simulink model "segway_control"  (R2022a)
settings: Solver=ode45  StartTime=0.0  StopTime=30  FixedStep=1e-3  RelTol=1e-3
PreLoadFcn:
  | preload
InitFcn:
  | init
  | preload
values from neighbouring files (symbols this model uses):
  A1 = [0 0   1 0 ... (first row only)    [plant.m]
  A2 = [0   1 ... (first row only)    [plant.m]
  B1 = [0 0 ... (first row only)    [plant.m]
  B2 = [0    0 ... (first row only)    [plant.m]
  C1 = [1 0 0 0 ... (first row only)    [plant.m]
  C2 = [1 0 ... (first row only)    [plant.m]
  D = 0.01    [params.m]
  D1 = zeros(4, 2)    [plant.m]
  D2 = zeros(2)    [plant.m]
  h = 0.21    [params.m]
  Jw = m * R^2 / 2    (= 0.0001458)    [params.m]
  Jwx = m * (3*R^2 + hw^2) / 12    (= 8.62333333333e-05)    [params.m]
  K = lqrd(s4.A, s4.B, QQ, RR, Ts)    [control.m]    (also in plant.m = W / (2 * R) * alpha)
  K_PWM = 8.087    [params.m]
  Kb = 0.468    [params.m]
  Kt = 0.317    [params.m]
  Lm = 0.0029    [params.m]
  m = 0.4    [params.m]
  M = 1.8    [params.m]
  R = 0.027    [params.m]
  Rm = 6.69    [params.m]
  W = 0.105    [params.m]
undefined symbols (not defined in the file or in its folder): X, Y, Z
libraries: sm_lib x17, nesl_utility x13, simulink_extras x7
settings Model: Creator=skakd  LastModifiedBy=skakd
settings SolverCC: ZeroCrossControl=EnableAll  ZeroCrossAlgorithm=Adaptive  EnableFixedStepZeroCrossing=on

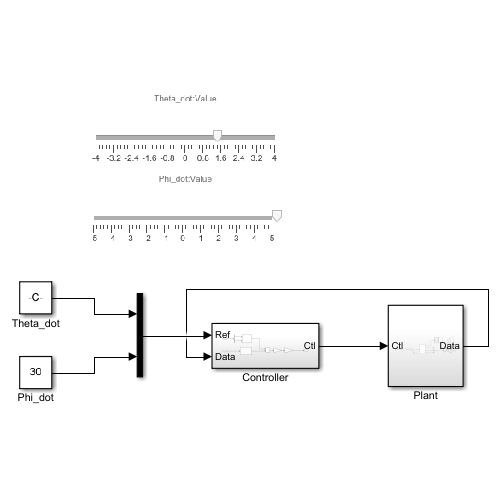
[thumbnail: Simulink's stored preview of the top-level diagram]
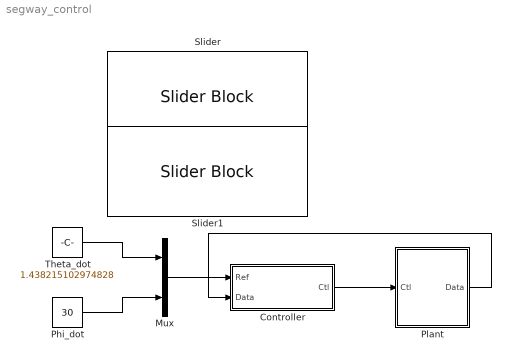
== system segway_control ==
  Controller : Subsystem
  Mux : Mux  Inputs=2
  Phi_dot : Constant  Value=30
  Plant : Subsystem
  Slider : SliderBlock  ScaleMin=-4  ScaleMax=4
  Slider1 : SliderBlock  ScaleMin=-5  ScaleMax=5
  Theta_dot : Constant  Value=1.438215102974828
  wires:
  Theta_dot/1 -> Mux/1
  Phi_dot/1 -> Mux/2
  Mux/1 -> Controller/1(Ref)
  Controller/1(Ctl) -> Plant/1(Ctl)
  Plant/1(Data) -> Controller/2(Data)

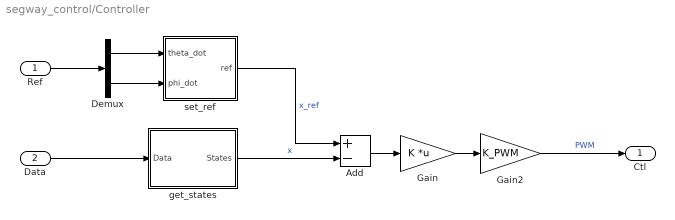
== system segway_control/Controller ==
  Ref : Inport
  Data : Inport  Port=2
  Add : Sum  Inputs=+-
  Demux : Demux  Outputs=2
  Gain : Gain  Gain=K  Multiplication=Matrix(K*u)
  Gain2 : Gain  Gain=K_PWM
  get_states : Subsystem
  set_ref : Subsystem
  Ctl : Outport  VectorParamsAs1DForOutWhenUnconnected=off
  wires:
  Gain2/1 -> Ctl/1  "PWM"
  Add/1 -> Gain/1
  set_ref/1(ref) -> Add/1  "x_ref"
  Gain/1 -> Gain2/1
  Ref/1 -> Demux/1
  Demux/1 -> set_ref/1(theta_dot)
  Demux/2 -> set_ref/2(phi_dot)
  get_states/1(States) -> Add/2  "x"
  Data/1 -> get_states/1(Data)

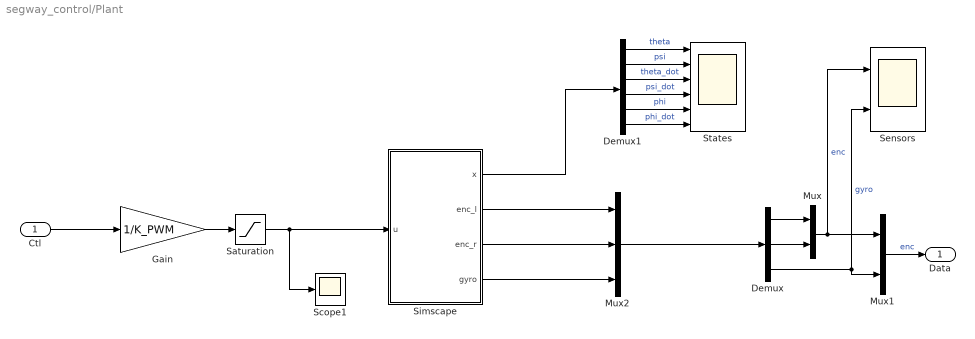
== system segway_control/Plant ==
  Ctl : Inport
  Demux : Demux  Outputs=3
  Demux1 : Demux  Outputs=6
  Gain : Gain  Gain=1/K_PWM
  Mux : Mux  Inputs=2
  Mux1 : Mux  Inputs=2
  Mux2 : Mux  Inputs=3
  Saturation : Saturate  UpperLimit=80  LowerLimit=-80
  Scope1 : Scope
  Sensors : Scope  NumInputPorts=2
  Simscape : Subsystem  Variant=on  VariantControl=Choice
  States : Scope  NumInputPorts=6
  Data : Outport
  wires:
  Mux2/1 -> Demux/1
  Demux/1 -> Mux/1
  Demux/2 -> Mux/2
  Mux/1 -> Mux1/1, Sensors/1  "enc"
  Demux/3 -> Mux1/2, Sensors/2  "gyro"
  Ctl/1 -> Gain/1
  Demux1/3 -> States/3  "theta_dot"
  Demux1/1 -> States/1  "theta"
  Demux1/4 -> States/4  "psi_dot"
  Demux1/6 -> States/6  "phi_dot"
  Demux1/2 -> States/2  "psi"
  Demux1/5 -> States/5  "phi"
  Gain/1 -> Saturation/1
  Saturation/1 -> Scope1/1, Simscape/1(u)
  Simscape/1(x) -> Demux1/1
  Simscape/2(enc_l) -> Mux2/1
  Simscape/3(enc_r) -> Mux2/2
  Simscape/4(gyro) -> Mux2/3
  Mux1/1 -> Data/1  "enc"

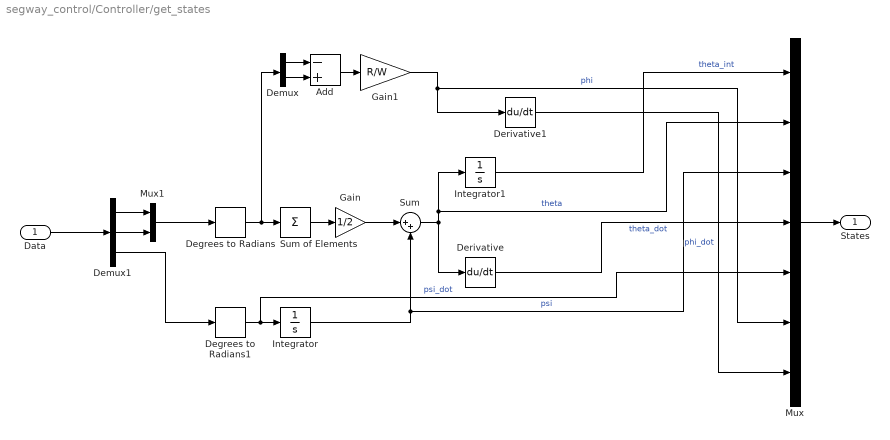
== system segway_control/Controller/get_states ==
  Data : Inport
  Add : Sum  Inputs=-+
  Degrees to Radians : simulink_extras/Transformations/Degrees to Radians
  Degrees to Radians1 : simulink_extras/Transformations/Degrees to Radians
  Demux : Demux  Outputs=2
  Demux1 : Demux  Outputs=3
  Derivative : Derivative
  Derivative1 : Derivative
  Gain : Gain  Gain=1/2
  Gain1 : Gain  Gain=R/W
  Integrator : Integrator
  Integrator1 : Integrator
  Mux : Mux  Inputs=7
  Mux1 : Mux  Inputs=2
  Sum : Sum  Inputs=|++
  Sum of Elements : Sum  Inputs=+
  States : Outport  VectorParamsAs1DForOutWhenUnconnected=off
  wires:
  Gain/1 -> Sum/1
  Degrees to Radians/1 -> Demux/1, Sum of Elements/1
  Integrator/1 -> Mux/3, Sum/2  "psi"
  Data/1 -> Demux1/1
  Mux1/1 -> Degrees to Radians/1
  Sum/1 -> Mux/2, Integrator1/1, Derivative/1  "theta"
  Derivative/1 -> Mux/4  "theta_dot"
  Sum of Elements/1 -> Gain/1
  Degrees to Radians1/1 -> Mux/5, Integrator/1  "psi_dot"
  Integrator1/1 -> Mux/1  "theta_int"
  Demux/1 -> Add/1
  Demux/2 -> Add/2
  Add/1 -> Gain1/1
  Gain1/1 -> Mux/6, Derivative1/1  "phi"
  Derivative1/1 -> Mux/7  "phi_dot"
  Mux/1 -> States/1
  Demux1/1 -> Mux1/1
  Demux1/2 -> Mux1/2
  Demux1/3 -> Degrees to Radians1/1

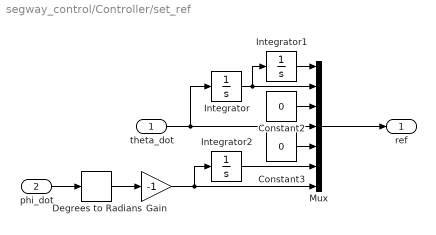
== system segway_control/Controller/set_ref ==
  theta_dot : Inport
  phi_dot : Inport  Port=2
  Constant2 : Constant  Value=0
  Constant3 : Constant  Value=0
  Degrees to Radians : simulink_extras/Transformations/Degrees to Radians
  Gain : Gain  Gain=-1
  Integrator : Integrator
  Integrator1 : Integrator
  Integrator2 : Integrator
  Mux : Mux  Inputs=7
  ref : Outport  VectorParamsAs1DForOutWhenUnconnected=off
  wires:
  Constant2/1 -> Mux/3
  Constant3/1 -> Mux/5
  Mux/1 -> ref/1
  Integrator/1 -> Integrator1/1, Mux/2
  phi_dot/1 -> Degrees to Radians/1
  Integrator2/1 -> Mux/6
  Integrator1/1 -> Mux/1
  theta_dot/1 -> Integrator/1, Mux/4
  Degrees to Radians/1 -> Gain/1
  Gain/1 -> Integrator2/1, Mux/7

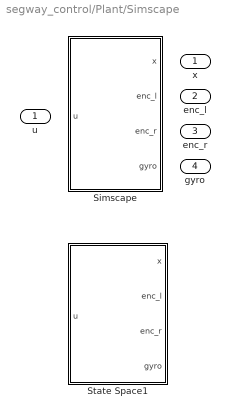
== system segway_control/Plant/Simscape ==
  u : Inport
  Simscape : Subsystem  VariantControl=(default)
  State Space1 : Subsystem  VariantControl=is_simscape == 0
  x : Outport
  enc_l : Outport  Port=2
  enc_r : Outport  Port=3
  gyro : Outport  Port=4

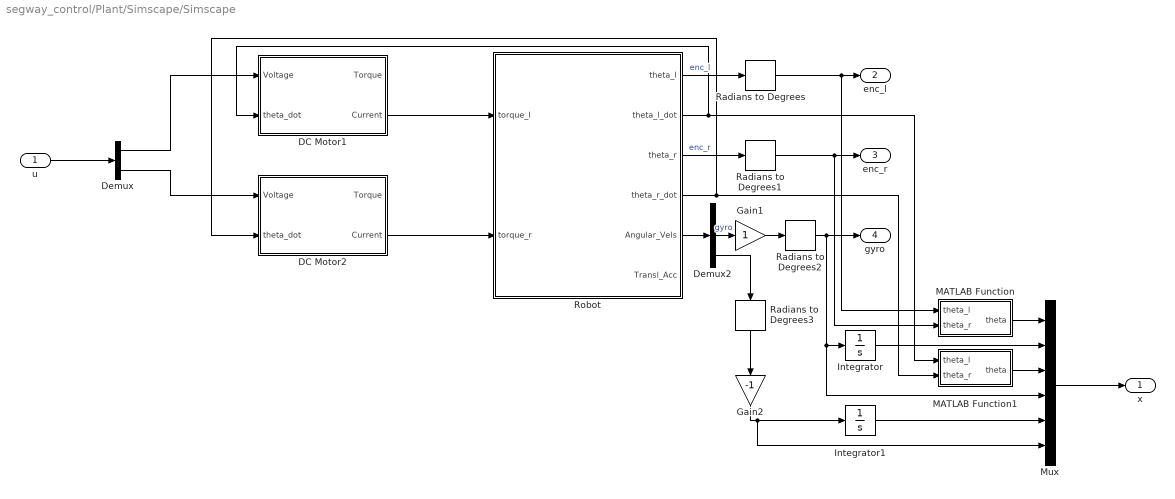
== system segway_control/Plant/Simscape/Simscape ==
  u : Inport
  DC Motor1 : Subsystem
  DC Motor2 : Subsystem
  Demux : Demux  Outputs=2
  Demux2 : Demux  Outputs=3
  Gain1 : Gain
  Gain2 : Gain  Gain=-1
  Integrator : Integrator
  Integrator1 : Integrator
  MATLAB Function : MATLAB Function  TreatAsAtomicUnit=on
  MATLAB Function1 : MATLAB Function  TreatAsAtomicUnit=on
  Mux : Mux  Inputs=6
  Radians to Degrees{,1..3} (4 alike) : simulink_extras/Transformations/Radians to Degrees
  Robot : Subsystem
  x : Outport
  enc_l : Outport  Port=2
  enc_r : Outport  Port=3
  gyro : Outport  Port=4
  wires:
  Robot/5(Angular_Vels) -> Demux2/1
  Demux2/2 -> Gain1/1  "gyro"
  Radians to Degrees1/1 -> MATLAB Function/2(theta_r), enc_r/1
  Robot/3(theta_r) -> Radians to Degrees1/1  "enc_r"
  Radians to Degrees/1 -> MATLAB Function/1(theta_l), enc_l/1
  Robot/1(theta_l) -> Radians to Degrees/1  "enc_l"
  Radians to Degrees2/1 -> gyro/1, Mux/4, Integrator/1
  u/1 -> Demux/1
  Mux/1 -> x/1
  Integrator/1 -> Mux/2
  Demux2/3 -> Radians to Degrees3/1
  Integrator1/1 -> Mux/5
  MATLAB Function/1(theta) -> Mux/1
  MATLAB Function1/1(theta) -> Mux/3
  Robot/2(theta_l_dot) -> DC Motor1/2(theta_dot), MATLAB Function1/1(theta_l)
  Robot/4(theta_r_dot) -> DC Motor2/2(theta_dot), MATLAB Function1/2(theta_r)
  Gain1/1 -> Radians to Degrees2/1
  Demux/1 -> DC Motor1/1(Voltage)
  Demux/2 -> DC Motor2/1(Voltage)
  Gain2/1 -> Integrator1/1, Mux/6
  DC Motor1/2(Current) -> Robot/1(torque_l)
  DC Motor2/2(Current) -> Robot/2(torque_r)
  Radians to Degrees3/1 -> Gain2/1

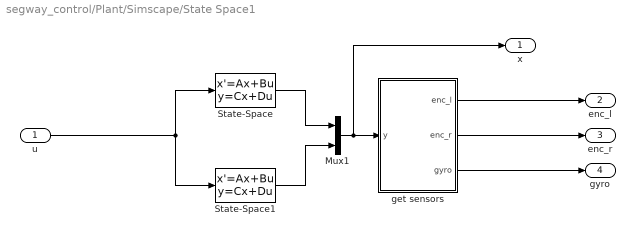
== system segway_control/Plant/Simscape/State Space1 ==
  u : Inport
  Mux1 : Mux  Inputs=2
  State-Space : StateSpace  A=A1  B=B1  C=C1  D=D1  InitialCondition=0
  State-Space1 : StateSpace  A=A2  B=B2  C=C2  D=D2  InitialCondition=0
  get sensors : MATLAB Function  TreatAsAtomicUnit=on
  x : Outport
  enc_l : Outport  Port=2
  enc_r : Outport  Port=3
  gyro : Outport  Port=4
  wires:
  get sensors/3(gyro) -> gyro/1
  get sensors/2(enc_r) -> enc_r/1
  State-Space1/1 -> Mux1/2
  u/1 -> State-Space1/1, State-Space/1
  Mux1/1 -> get sensors/1(y), x/1
  State-Space/1 -> Mux1/1
  get sensors/1(enc_l) -> enc_l/1

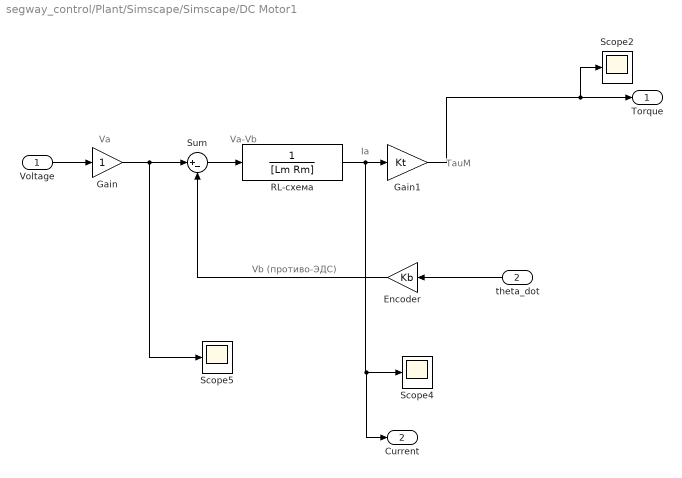
== system segway_control/Plant/Simscape/Simscape/DC Motor1 ==
  note: Va
  note: Va-Vb
  note: Vb (противо-ЭДС)
  note: Ia
  note: TauM
  Voltage : Inport
  theta_dot : Inport  Port=2
  Encoder : Gain  Gain=Kb
  Gain : Gain
  Gain1 : Gain  Gain=Kt
  RL-схема : TransferFcn  Denominator=[Lm Rm]
  Scope2 : Scope
  Scope4 : Scope
  Scope5 : Scope
  Sum : Sum  Inputs=|+-
  Torque : Outport
  Current : Outport  Port=2
  wires:
  Voltage/1 -> Gain/1
  Encoder/1 -> Sum/2
  Sum/1 -> RL-схема/1
  RL-схема/1 -> Gain1/1, Scope4/1, Current/1
  Gain/1 -> Sum/1, Scope5/1
  Gain1/1 -> Scope2/1, Torque/1
  theta_dot/1 -> Encoder/1

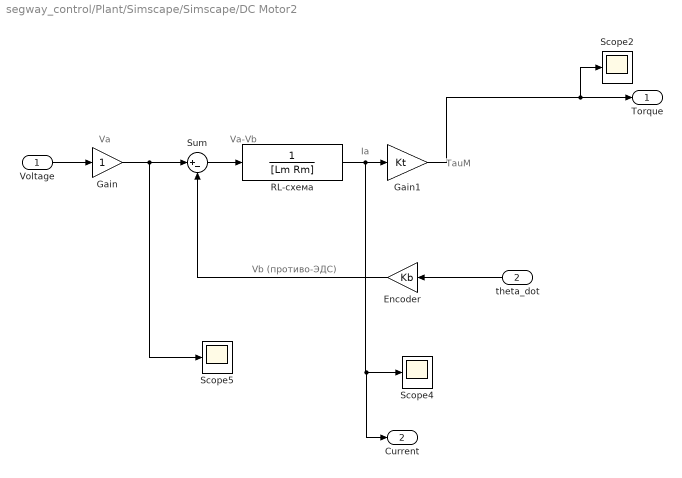
== system segway_control/Plant/Simscape/Simscape/DC Motor2 ==
  note: TauM
  note: Ia
  note: Vb (противо-ЭДС)
  note: Va-Vb
  note: Va
  Voltage : Inport
  theta_dot : Inport  Port=2
  Encoder : Gain  Gain=Kb
  Gain : Gain
  Gain1 : Gain  Gain=Kt
  RL-схема : TransferFcn  Denominator=[Lm Rm]
  Scope2 : Scope
  Scope4 : Scope
  Scope5 : Scope
  Sum : Sum  Inputs=|+-
  Torque : Outport
  Current : Outport  Port=2
  wires:
  theta_dot/1 -> Encoder/1
  Gain1/1 -> Torque/1, Scope2/1
  Gain/1 -> Scope5/1, Sum/1
  RL-схема/1 -> Current/1, Scope4/1, Gain1/1
  Sum/1 -> RL-схема/1
  Encoder/1 -> Sum/2
  Voltage/1 -> Gain/1

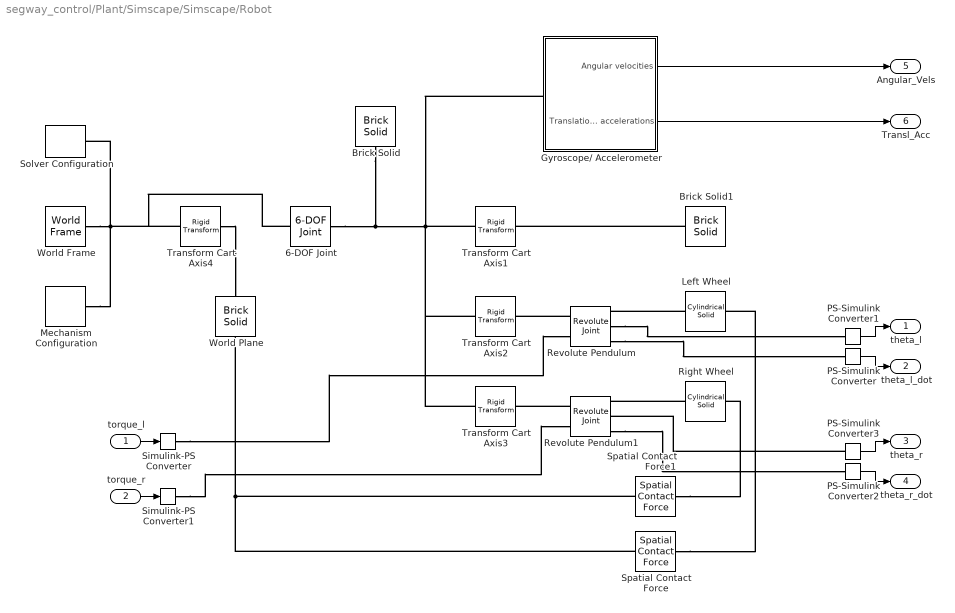
== system segway_control/Plant/Simscape/Simscape/Robot ==
  torque_l : Inport
  torque_r : Inport  Port=2
  6-DOF Joint : sm_lib/Joints/6-DOF Joint  JointMode=Normal  SenseConstraintForce=off  SenseConstraintForceX=off  SenseConstraintForceY=off  SenseConstraintForceZ=off  SenseConstraintTorque=off  SenseConstraintTorqueX=off  SenseConstraintTorqueY=off  SenseConstraintTorqueZ=off  SenseTotalForce=off  SenseTotalForceX=off  SenseTotalForceY=off  SenseTotalForceZ=off  SenseTotalTorque=off  SenseTotalTorqueX=off  SenseTotalTorqueY=off  SenseTotalTorqueZ=off  CompositeWrenchDir=FollowerOnBase  CompositeWrenchFrame=BaseFrame  PxEquilibriumPosition=0  PxEquilibriumPositionUnits=m  PxSpringStiffness=0  PxSpringStiffnessUnits=N/m  PxDampingCoefficient=0  PxDampingCoefficientUnits=N/(m/s)  PxTorqueActuationMode=NoTorque  PxMotionActuationMode=ComputedMotion  PxSensePosition=off  PxSenseVelocity=off  PxSenseAcceleration=off  PxSenseTorqueForce=off  PxSenseLowerLimitTorqueForce=off  PxSenseUpperLimitTorqueForce=off  PxLowerLimitSpecify=off  PxLowerLimitBound=-1  PxLowerLimitBoundUnits=m  PxLowerLimitStiffness=1e6  PxLowerLimitStiffnessUnits=N/m  PxLowerLimitDamping=1e3  PxLowerLimitDampingUnits=N/(m/s)  PxLowerLimitTransitionRegionWidth=1e-4  PxLowerLimitTransitionRegionWidthUnits=m  PxUpperLimitSpecify=off  PxUpperLimitBound=1  PxUpperLimitBoundUnits=m  PxUpperLimitStiffness=1e6  PxUpperLimitStiffnessUnits=N/m  PxUpperLimitDamping=1e3  PxUpperLimitDampingUnits=N/(m/s)  PxUpperLimitTransitionRegionWidth=1e-4  PxUpperLimitTransitionRegionWidthUnits=m  PxPositionTargetSpecify=off  PxPositionTargetPriority=High  PxPositionTargetValue=0  PxPositionTargetValueUnits=m  PxVelocityTargetSpecify=off  PxVelocityTargetPriority=High  PxVelocityTargetValue=0  PxVelocityTargetValueUnits=m/s  PyEquilibriumPosition=0  PyEquilibriumPositionUnits=m  PySpringStiffness=0  PySpringStiffnessUnits=N/m  PyDampingCoefficient=0  PyDampingCoefficientUnits=N/(m/s)  PyTorqueActuationMode=NoTorque  PyMotionActuationMode=ComputedMotion  PySensePosition=off  PySenseVelocity=off  PySenseAcceleration=off  PySenseTorqueForce=off  PySenseLowerLimitTorqueForce=off  PySenseUpperLimitTorqueForce=off  PyLowerLimitSpecify=off  PyLowerLimitBound=-1  PyLowerLimitBoundUnits=m  PyLowerLimitStiffness=1e6  PyLowerLimitStiffnessUnits=N/m  PyLowerLimitDamping=1e3  PyLowerLimitDampingUnits=N/(m/s)  PyLowerLimitTransitionRegionWidth=1e-4  PyLowerLimitTransitionRegionWidthUnits=m  PyUpperLimitSpecify=off  PyUpperLimitBound=1  PyUpperLimitBoundUnits=m  PyUpperLimitStiffness=1e6  PyUpperLimitStiffnessUnits=N/m  PyUpperLimitDamping=1e3  PyUpperLimitDampingUnits=N/(m/s)  PyUpperLimitTransitionRegionWidth=1e-4  PyUpperLimitTransitionRegionWidthUnits=m  PyPositionTargetSpecify=off  PyPositionTargetPriority=High  PyPositionTargetValue=0  PyPositionTargetValueUnits=m  PyVelocityTargetSpecify=off  PyVelocityTargetPriority=High  PyVelocityTargetValue=0  PyVelocityTargetValueUnits=m/s  PzEquilibriumPosition=0  PzEquilibriumPositionUnits=m  PzSpringStiffness=0  PzSpringStiffnessUnits=N/m  PzDampingCoefficient=0  PzDampingCoefficientUnits=N/(m/s)  PzTorqueActuationMode=NoTorque  PzMotionActuationMode=ComputedMotion  PzSensePosition=off  PzSenseVelocity=off  PzSenseAcceleration=off  PzSenseTorqueForce=off  PzSenseLowerLimitTorqueForce=off  PzSenseUpperLimitTorqueForce=off  PzLowerLimitSpecify=off  PzLowerLimitBound=-1  PzLowerLimitBoundUnits=m  PzLowerLimitStiffness=1e6  PzLowerLimitStiffnessUnits=N/m  PzLowerLimitDamping=1e3  PzLowerLimitDampingUnits=N/(m/s)  PzLowerLimitTransitionRegionWidth=1e-4  PzLowerLimitTransitionRegionWidthUnits=m  PzUpperLimitSpecify=off  PzUpperLimitBound=1  PzUpperLimitBoundUnits=m  PzUpperLimitStiffness=1e6  PzUpperLimitStiffnessUnits=N/m  PzUpperLimitDamping=1e3  PzUpperLimitDampingUnits=N/(m/s)  PzUpperLimitTransitionRegionWidth=1e-4  PzUpperLimitTransitionRegionWidthUnits=m  PzPositionTargetSpecify=on  PzPositionTargetPriority=High  PzPositionTargetValue=R+0.025  PzPositionTargetValueUnits=m  PzVelocityTargetSpecify=off  PzVelocityTargetPriority=High  PzVelocityTargetValue=0  PzVelocityTargetValueUnits=m/s  SphDefPosRotationMethod=None  SphDefPosRotationAngleUnits=deg  SphDefPosRotationStandardAxis=+Z  SphDefPosRotationAngle=0.0  SphDefPosRotationArbitraryAxis=[0 0 1]  SphDefPosFollAlignAxisA=+X  SphDefPosBaseAlignAxisA=+Y  SphDefPosFollAlignAxisB=+Y  SphDefPosBaseAlignAxisB=+Z  SphDefPosRotationSequenceAxes=FollowerAxes  SphDefPosRotationSequence=XYX  SphDefPosRotationSequenceAngles=[0 0 0]  SphDefPosRotationSequenceAnglesUnits=deg  SphDefPosRotationMatrix=[1 0 0; 0 1 0; 0 0 1]  SphEqPosRotationMethod=None  SphEqPosRotationAngleUnits=deg  SphEqPosRotationStandardAxis=+Z  SphEqPosRotationAngle=0.0  SphEqPosRotationArbitraryAxis=[0 0 1]  SphEqPosFollAlignAxisA=+X  SphEqPosBaseAlignAxisA=+Y  SphEqPosFollAlignAxisB=+Y  SphEqPosBaseAlignAxisB=+Z  SphEqPosRotationSequenceAxes=FollowerAxes  SphEqPosRotationSequence=XYX  SphEqPosRotationSequenceAngles=[0 0 0]  SphEqPosRotationSequenceAnglesUnits=deg  SphEqPosRotationMatrix=[1 0 0; 0 1 0; 0 0 1]  SphSpringStiffness=0  SphSpringStiffnessUnits=N*m/deg  SphDampingCoefficient=0  SphDampingCoefficientUnits=N*m/(deg/s)  SphActuateTorqueX=off  SphActuateTorqueY=off  SphActuateTorqueZ=off  SphActuateTorque=off  SphTorqueActuationMode=NoTorque  SphMotionActuationMode=ComputedMotion  SphActuationFrame=BaseFrame  SphSensePosition=off  SphSenseVelocityX=off  SphSenseVelocityY=off  SphSenseVelocityZ=off  SphSenseVelocity=off  SphSenseAccelerationX=off  SphSenseAccelerationY=off  SphSenseAccelerationZ=off  SphSenseAcceleration=off  SphSenseTorqueX=off  SphSenseTorqueY=off  SphSenseTorqueZ=off  SphSenseTorqueForce=off  SphSenseLowerLimitTorqueMag=off  SphSenseUpperLimitTorqueMag=off  SphSensingFrame=BaseFrame  SphLowerLimitSpecify=off  SphLowerLimitBound=15  SphLowerLimitBoundUnits=deg  SphLowerLimitStiffness=1e4  SphLowerLimitStiffnessUnits=N*m/deg  SphLowerLimitDamping=10  SphLowerLimitDampingUnits=N*m/(deg/s)  SphLowerLimitTransitionRegionWidth=0.1  SphLowerLimitTransitionRegionWidthUnits=deg  SphUpperLimitSpecify=off  SphUpperLimitBound=45  SphUpperLimitBoundUnits=deg  SphUpperLimitStiffness=1e4  SphUpperLimitStiffnessUnits=N*m/deg  SphUpperLimitDamping=10  SphUpperLimitDampingUnits=N*m/(deg/s)  SphUpperLimitTransitionRegionWidth=0.1  SphUpperLimitTransitionRegionWidthUnits=deg  SphPositionTargetRotationMethod=None  SphPositionTargetRotationAngleUnits=deg  SphPositionTargetRotationStandardAxis=+Z  SphPositionTargetRotationAngle=0.0  SphPositionTargetRotationArbitraryAxis=[0 0 1]  SphPositionTargetFollAlignAxisA=+X  SphPositionTargetBaseAlignAxisA=+Y  SphPositionTargetFollAlignAxisB=+Y  SphPositionTargetBaseAlignAxisB=+Z  SphPositionTargetRotationSequenceAxes=FollowerAxes  SphPositionTargetRotationSequence=XYX  SphPositionTargetRotationSequenceAngles=[0 0 0]  SphPositionTargetRotationSequenceAnglesUnits=deg  SphPositionTargetRotationMatrix=[1 0 0; 0 1 0; 0 0 1]  SphPositionTargetSpecify=off  SphPositionTargetPriority=High  SphVelocityTargetValue=[0 0 0]  SphVelocityTargetValueUnits=deg/s  SphVelocityTargetSpecify=off  SphVelocityTargetPriority=High  SphVelocityTargetInFollowerFrame=on
  Brick Solid : sm_lib/Body Elements/Brick Solid  GraphicAmbientColor=[0.15 0.15 0.15 1.0]  BasedOnType=Density  BrickDimensions=[0.01 W 0.01]  BrickDimensionUnits=m  CenterOfMass=[0 0 0]  CenterOfMassUnits=m  GraphicDiffuseColor=[0.5 0.5 0.5]  Density=10  DensityUnits=kg/m^3  DoExposeReferenceFrame=on  GraphicEmissiveColor=[0.0 0.0 0.0 1.0]  ExportEntireGeometry=off  SerializedFrames=<Frames/>  MarkerShape=Sphere  MarkerSize=10  GraphicType=FromGeometry  InertiaType=CalculateFromGeometry  Mass=10  MassUnits=kg  MomentsOfInertia=[1 1 1]  MomentsOfInertiaUnits=kg*m^2  GraphicOpacity=1.0  ProductsOfInertia=[0 0 0]  ProductsOfInertiaUnits=kg*m^2  GraphicShininess=75  GraphicSpecularColor=[0.5 0.5 0.5 1.0]  GraphicVisPropType=SimpleVisualProperties
  Brick Solid1 : sm_lib/Body Elements/Brick Solid  GraphicAmbientColor=[0.15 0.15 0.15 1.0]  BasedOnType=Mass  BrickDimensions=[D W h]  BrickDimensionUnits=m  CenterOfMass=[0 0 0]  CenterOfMassUnits=m  GraphicDiffuseColor=[1.0 1.0 0.0]  Density=40000  DensityUnits=kg/m^3  DoExposeReferenceFrame=on  GraphicEmissiveColor=[0.0 0.0 0.0 1.0]  ExportEntireGeometry=on  SerializedFrames=<Frames/>  MarkerShape=Sphere  MarkerSize=10  GraphicType=FromGeometry  InertiaType=CalculateFromGeometry  Mass=M  MassUnits=kg  MomentsOfInertia=[1 1 1]  MomentsOfInertiaUnits=kg*m^2  GraphicOpacity=1.0  ProductsOfInertia=[0 0 0]  ProductsOfInertiaUnits=kg*m^2  GraphicShininess=75  GraphicSpecularColor=[0.5 0.5 0.5 1.0]  GraphicVisPropType=SimpleVisualProperties
  Gyroscope/ Accelerometer : Subsystem
  Left Wheel : sm_lib/Body Elements/Cylindrical Solid  GraphicAmbientColor=[0.15 0.15 0.15 1.0]  BasedOnType=Mass  CenterOfMass=[0 0 0]  CenterOfMassUnits=m  GraphicDiffuseColor=[0.2 0.2 0.2]  CylinderLength=0.02  CylinderLengthUnits=m  CylinderRadius=R  CylinderRadiusUnits=m  Density=5000  DensityUnits=kg/m^3  DoExposeReferenceFrame=on  GraphicEmissiveColor=[0.0 0.0 0.0 1.0]  ExportEntireGeometry=on  SerializedFrames=<Frames/>  MarkerShape=Sphere  MarkerSize=10  GraphicType=FromGeometry  InertiaType=CalculateFromGeometry  Mass=m  MassUnits=kg  MomentsOfInertia=[0 0 Jw]  MomentsOfInertiaUnits=kg*m^2  GraphicOpacity=1.0  ProductsOfInertia=[0 0 0]  ProductsOfInertiaUnits=kg*m^2  GraphicShininess=75  GraphicSpecularColor=[0.5 0.5 0.5 1.0]  GraphicVisPropType=SimpleVisualProperties
  Mechanism Configuration : sm_lib/Utilities/Mechanism Configuration  UniformGravity=Constant  GravityVector=[0 0 -9.80665]  GravityUnits=m/s^2  LinearizationDelta=0.001  JointModeTransitionNonlinearIterations=2
  PS-Simulink Converter{,1..3} (4 alike) : nesl_utility/PS-Simulink Converter  PhysicalDomain=network_engine_domain  SubClassName=ps_output  LeftPortType=input  RightPortType=output  PseudoPeriodic=off  Frequencies=[]  VectorFormat=inherit  Unit=inherit  AffineConversion=off
      settings: SourceProductBaseCode=SS,PW,VE
  Revolute Pendulum : sm_lib/Joints/Revolute Joint  JointMode=Normal  SenseConstraintForce=off  SenseConstraintForceX=off  SenseConstraintForceY=off  SenseConstraintForceZ=off  SenseConstraintTorque=off  SenseConstraintTorqueX=off  SenseConstraintTorqueY=off  SenseConstraintTorqueZ=off  SenseTotalForce=off  SenseTotalForceX=off  SenseTotalForceY=off  SenseTotalForceZ=off  SenseTotalTorque=off  SenseTotalTorqueX=off  SenseTotalTorqueY=off  SenseTotalTorqueZ=off  CompositeWrenchDir=FollowerOnBase  CompositeWrenchFrame=BaseFrame  EquilibriumPosition=0  EquilibriumPositionUnits=deg  SpringStiffness=0  SpringStiffnessUnits=N*m/deg  DampingCoefficient=fm  DampingCoefficientUnits=N*m/(deg/s)  TorqueActuationMode=InputTorque  MotionActuationMode=ComputedMotion  SensePosition=on  SenseVelocity=on  SenseAcceleration=off  SenseTorqueForce=off  SenseLowerLimitTorqueForce=off  SenseUpperLimitTorqueForce=off  LowerLimitSpecify=off  LowerLimitBound=-90  LowerLimitBoundUnits=deg  LowerLimitStiffness=1e4  LowerLimitStiffnessUnits=N*m/deg  LowerLimitDamping=10  LowerLimitDampingUnits=N*m/(deg/s)  LowerLimitTransitionRegionWidth=0.1  LowerLimitTransitionRegionWidthUnits=deg  UpperLimitSpecify=off  UpperLimitBound=90  UpperLimitBoundUnits=deg  UpperLimitStiffness=1e4  UpperLimitStiffnessUnits=N*m/deg  UpperLimitDamping=10  UpperLimitDampingUnits=N*m/(deg/s)  UpperLimitTransitionRegionWidth=0.1  UpperLimitTransitionRegionWidthUnits=deg  PositionTargetSpecify=off  PositionTargetPriority=High  PositionTargetValue=0  PositionTargetValueUnits=deg  VelocityTargetSpecify=off  VelocityTargetPriority=High  VelocityTargetValue=0  VelocityTargetValueUnits=deg/s
  Revolute Pendulum1 : sm_lib/Joints/Revolute Joint  JointMode=Normal  SenseConstraintForce=off  SenseConstraintForceX=off  SenseConstraintForceY=off  SenseConstraintForceZ=off  SenseConstraintTorque=off  SenseConstraintTorqueX=off  SenseConstraintTorqueY=off  SenseConstraintTorqueZ=off  SenseTotalForce=off  SenseTotalForceX=off  SenseTotalForceY=off  SenseTotalForceZ=off  SenseTotalTorque=off  SenseTotalTorqueX=off  SenseTotalTorqueY=off  SenseTotalTorqueZ=off  CompositeWrenchDir=FollowerOnBase  CompositeWrenchFrame=BaseFrame  EquilibriumPosition=0  EquilibriumPositionUnits=deg  SpringStiffness=0  SpringStiffnessUnits=N*m/deg  DampingCoefficient=fm  DampingCoefficientUnits=N*m/(deg/s)  TorqueActuationMode=InputTorque  MotionActuationMode=ComputedMotion  SensePosition=on  SenseVelocity=on  SenseAcceleration=off  SenseTorqueForce=off  SenseLowerLimitTorqueForce=off  SenseUpperLimitTorqueForce=off  LowerLimitSpecify=off  LowerLimitBound=-90  LowerLimitBoundUnits=deg  LowerLimitStiffness=1e4  LowerLimitStiffnessUnits=N*m/deg  LowerLimitDamping=10  LowerLimitDampingUnits=N*m/(deg/s)  LowerLimitTransitionRegionWidth=0.1  LowerLimitTransitionRegionWidthUnits=deg  UpperLimitSpecify=off  UpperLimitBound=90  UpperLimitBoundUnits=deg  UpperLimitStiffness=1e4  UpperLimitStiffnessUnits=N*m/deg  UpperLimitDamping=10  UpperLimitDampingUnits=N*m/(deg/s)  UpperLimitTransitionRegionWidth=0.1  UpperLimitTransitionRegionWidthUnits=deg  PositionTargetSpecify=off  PositionTargetPriority=High  PositionTargetValue=0  PositionTargetValueUnits=deg  VelocityTargetSpecify=off  VelocityTargetPriority=High  VelocityTargetValue=0  VelocityTargetValueUnits=deg/s
  Right Wheel : sm_lib/Body Elements/Cylindrical Solid  GraphicAmbientColor=[0.15 0.15 0.15 1.0]  BasedOnType=Mass  CenterOfMass=[0 0 0]  CenterOfMassUnits=m  GraphicDiffuseColor=[0.2 0.2 0.2]  CylinderLength=hw  CylinderLengthUnits=m  CylinderRadius=R  CylinderRadiusUnits=m  Density=1000  DensityUnits=kg/m^3  DoExposeReferenceFrame=on  GraphicEmissiveColor=[0.0 0.0 0.0 1.0]  ExportEntireGeometry=on  SerializedFrames=<Frames/>  MarkerShape=Sphere  MarkerSize=10  GraphicType=FromGeometry  InertiaType=CalculateFromGeometry  Mass=m  MassUnits=kg  MomentsOfInertia=[Jwx Jwx Jw]  MomentsOfInertiaUnits=kg*m^2  GraphicOpacity=1.0  ProductsOfInertia=[0 0 0]  ProductsOfInertiaUnits=kg*m^2  GraphicShininess=75  GraphicSpecularColor=[0.5 0.5 0.5 1.0]  GraphicVisPropType=SimpleVisualProperties
  Simulink-PS Converter : nesl_utility/Simulink-PS Converter  PhysicalDomain=network_engine_domain  SubClassName=ps_input  LeftPortType=input  RightPortType=output  PseudoPeriodic=off  Frequencies=[]  NoiseDistribution=none  NoiseParameters=[]  Unit=1  AffineConversion=off  FilteringAndDerivatives=provide  SimscapeFilterOrder=1  InputFilterTimeConstant=0.001  UdotUserProvided=0
      settings: SourceProductBaseCode=SS,PW,VE
  Simulink-PS Converter1 : nesl_utility/Simulink-PS Converter  PhysicalDomain=network_engine_domain  SubClassName=ps_input  LeftPortType=input  RightPortType=output  PseudoPeriodic=off  Frequencies=[]  NoiseDistribution=none  NoiseParameters=[]  Unit=1  AffineConversion=off  FilteringAndDerivatives=provide  SimscapeFilterOrder=1  InputFilterTimeConstant=0.001  UdotUserProvided=0
      settings: SourceProductBaseCode=SS,PW,VE
  Solver Configuration : nesl_utility/Solver Configuration  PhysicalDomain=network_engine_domain  SubClassName=solver  LeftPortType=input  RightPortType=generic  Tones=[]  Harmonics=[]  SimulateNoise=off  Profile=off  UseLocalSampling=off  EnableSwitchedLinearOptims=on  FrequencyDomain=off  UseCCode=off  RelTol=0.001  AbsTol=1e-06  MinStep=1e-09  ToWorkspace=off  RevertToSquareIcSolve=off  NumHomotopyIterations=100  PhasorMode=off  PhasorModeNumHarmonics=1  IndexReductionMethod=DerivativeReplacement  DoDC=off  ResidualTolerance=1e-09  UseLocalSolver=off  LocalSolverChoice=NE_BACKWARD_EULER_ADVANCER  LocalSolverSampleTime=0.001  DoFixedCost=off  MaxNonlinIter=3  MaxModeIter=2  ComputeImpulses=off  ImpulseIterations=2  LinearAlgebra=Sparse  LinearAlgebraNumThread=0  EquationFormulation=NE_TIME_EF  DelaysMemoryBudget=1024  AutomaticFiltering=on  FilteringTimeConstant=0.001  PartitionStorageMethod=AS_NEEDED  PartitionMemoryBudget=1024  PartitionMethod=FAST
      settings: SourceProductBaseCode=SS,PW,VE
  Spatial Contact Force : sm_lib/Forces and Torques/Spatial Contact Force  SenseContactBaseRotation=off  SenseContactBaseTranslation=off  CoefficientOfDynamicFriction=1  CoefficientOfStaticFriction=1  NormalDamping=1e3  NormalDampingUnits=N/(m/s)  SenseContactSignal=off  NormalStiffness=1e6  NormalStiffnessUnits=N/m  FrictionalCriticalVelocity=1e-2  FrictionalCriticalVelocityUnits=m/s  ZeroCrossDetectContactStartAndEnd=off  SenseContactFollowerRotation=off  SenseContactFollowerTranslation=off  FrictionType=SmoothStickSlip  SenseFrictionalForceMagnitude=off  SenseNormalForceMagnitude=off  NormalForceType=SmoothSpringDamper  SenseNormalVelocity=off  SenseSeparationDistance=off  SenseTangentialVelocity=off  NormalTransitionRegionWidth=1e-4  NormalTransitionRegionWidthUnits=m
  Spatial Contact Force1 : sm_lib/Forces and Torques/Spatial Contact Force  SenseContactBaseRotation=off  SenseContactBaseTranslation=off  CoefficientOfDynamicFriction=1  CoefficientOfStaticFriction=1  NormalDamping=1e3  NormalDampingUnits=N/(m/s)  SenseContactSignal=off  NormalStiffness=1e6  NormalStiffnessUnits=N/m  FrictionalCriticalVelocity=1e-2  FrictionalCriticalVelocityUnits=m/s  ZeroCrossDetectContactStartAndEnd=off  SenseContactFollowerRotation=off  SenseContactFollowerTranslation=off  FrictionType=SmoothStickSlip  SenseFrictionalForceMagnitude=off  SenseNormalForceMagnitude=off  NormalForceType=SmoothSpringDamper  SenseNormalVelocity=off  SenseSeparationDistance=off  SenseTangentialVelocity=off  NormalTransitionRegionWidth=1e-4  NormalTransitionRegionWidthUnits=m
  Transform Cart Axis1 : sm_lib/Frames and Transforms/Rigid Transform  TranslationMethod=StandardAxis  TranslationStandardOffset=L  TranslationLengthUnit=m  TranslationStandardAxis=+Z  TranslationCartesianOffset=[0 0 0]  TranslationROffset=0  TranslationROffsetUnits=m  TranslationZOffset=0  TranslationZOffsetUnits=m  TranslationThetaOffset=0  TranslationThetaOffsetUnits=deg  RotationMethod=None  RotationAngleUnits=deg  RotationStandardAxis=+Y  RotationAngle=90  RotationArbitraryAxis=[0 0 1]  FollAlignAxisA=+X  BaseAlignAxisA=+Y  FollAlignAxisB=+Y  BaseAlignAxisB=+Z  RotationSequenceAxes=FollowerAxes  RotationSequence=XYX  RotationSequenceAngles=[0 0 0]  RotationSequenceAnglesUnits=deg  RotationMatrix=[1 0 0; 0 1 0; 0 0 1]
  Transform Cart Axis2 : sm_lib/Frames and Transforms/Rigid Transform  TranslationMethod=StandardAxis  TranslationStandardOffset=W/2  TranslationLengthUnit=m  TranslationStandardAxis=+Y  TranslationCartesianOffset=[0 W/2 0]  TranslationROffset=0  TranslationROffsetUnits=m  TranslationZOffset=0  TranslationZOffsetUnits=m  TranslationThetaOffset=0  TranslationThetaOffsetUnits=deg  RotationMethod=StandardAxis  RotationAngleUnits=deg  RotationStandardAxis=+X  RotationAngle=90  RotationArbitraryAxis=[0 0 1]  FollAlignAxisA=+X  BaseAlignAxisA=+Y  FollAlignAxisB=+Y  BaseAlignAxisB=+Z  RotationSequenceAxes=FollowerAxes  RotationSequence=XYX  RotationSequenceAngles=[0 0 0]  RotationSequenceAnglesUnits=deg  RotationMatrix=[1 0 0; 0 1 0; 0 0 1]
  Transform Cart Axis3 : sm_lib/Frames and Transforms/Rigid Transform  TranslationMethod=StandardAxis  TranslationStandardOffset=W/2  TranslationLengthUnit=m  TranslationStandardAxis=-Y  TranslationCartesianOffset=[0 0 0]  TranslationROffset=0  TranslationROffsetUnits=m  TranslationZOffset=0  TranslationZOffsetUnits=m  TranslationThetaOffset=0  TranslationThetaOffsetUnits=deg  RotationMethod=RotationSequence  RotationAngleUnits=deg  RotationStandardAxis=+X  RotationAngle=90  RotationArbitraryAxis=[0 0 1]  FollAlignAxisA=+X  BaseAlignAxisA=+Y  FollAlignAxisB=+Y  BaseAlignAxisB=+Z  RotationSequenceAxes=FollowerAxes  RotationSequence=XYX  RotationSequenceAngles=[90 0 0]  RotationSequenceAnglesUnits=deg  RotationMatrix=[1 0 0; 0 1 0; 0 0 1]
  Transform Cart Axis4 : sm_lib/Frames and Transforms/Rigid Transform  TranslationMethod=StandardAxis  TranslationStandardOffset=0  TranslationLengthUnit=m  TranslationStandardAxis=+Z  TranslationCartesianOffset=[0 0 0]  TranslationROffset=0  TranslationROffsetUnits=m  TranslationZOffset=0  TranslationZOffsetUnits=m  TranslationThetaOffset=0  TranslationThetaOffsetUnits=deg  RotationMethod=StandardAxis  RotationAngleUnits=deg  RotationStandardAxis=+Y  RotationAngle=0  RotationArbitraryAxis=[0 0 1]  FollAlignAxisA=+X  BaseAlignAxisA=+Y  FollAlignAxisB=+Y  BaseAlignAxisB=+Z  RotationSequenceAxes=FollowerAxes  RotationSequence=XYX  RotationSequenceAngles=[0 0 0]  RotationSequenceAnglesUnits=deg  RotationMatrix=[1 0 0; 0 1 0; 0 0 1]
  World Frame : sm_lib/Frames and Transforms/World Frame
  World Plane : sm_lib/Body Elements/Brick Solid  GraphicAmbientColor=[0.15 0.15 0.15 1.0]  BasedOnType=Density  BrickDimensions=[10 10 0.05]  BrickDimensionUnits=m  CenterOfMass=[0 0 0]  CenterOfMassUnits=m  GraphicDiffuseColor=[0.0 0.8 0.0]  Density=1000  DensityUnits=kg/m^3  DoExposeReferenceFrame=on  GraphicEmissiveColor=[0.0 0.0 0.0 1.0]  ExportEntireGeometry=on  SerializedFrames=<Frames/>  MarkerShape=Sphere  MarkerSize=10  GraphicType=FromGeometry  InertiaType=PointMass  Mass=0.1  MassUnits=kg  MomentsOfInertia=[1 1 1]  MomentsOfInertiaUnits=kg*m^2  GraphicOpacity=1.0  ProductsOfInertia=[0 0 0]  ProductsOfInertiaUnits=kg*m^2  GraphicShininess=75  GraphicSpecularColor=[0.5 0.5 0.5 1.0]  GraphicVisPropType=SimpleVisualProperties
  theta_l : Outport
  theta_l_dot : Outport  Port=2
  theta_r : Outport  Port=3
  theta_r_dot : Outport  Port=4
  Angular_Vels : Outport  Port=5
  Transl_Acc : Outport  Port=6
  wires:
  torque_l/1 -> Simulink-PS Converter/1
  torque_r/1 -> Simulink-PS Converter1/1
  PS-Simulink Converter1/1 -> theta_l/1
  PS-Simulink Converter/1 -> theta_l_dot/1
  PS-Simulink Converter2/1 -> theta_r_dot/1
  PS-Simulink Converter3/1 -> theta_r/1
  Gyroscope/ Accelerometer/1(Angular velocities) -> Angular_Vels/1
  Gyroscope/ Accelerometer/2(Translation accelerations) -> Transl_Acc/1
  connections:
  Revolute Pendulum/RConn2 -- PS-Simulink Converter1/LConn1
  Spatial Contact Force1/RConn1 -- Right Wheel/LConn1
  Simulink-PS Converter1/RConn1 -- Revolute Pendulum1/LConn2
  Brick Solid1/RConn1 -- Transform Cart Axis1/RConn1
  Spatial Contact Force/RConn1 -- Left Wheel/LConn1
  Revolute Pendulum1/LConn1 -- Transform Cart Axis3/RConn1
  Revolute Pendulum/LConn1 -- Transform Cart Axis2/RConn1
  6-DOF Joint/RConn1 -- Brick Solid/RConn1 -- Transform Cart Axis1/LConn1 -- Transform Cart Axis3/LConn1 -- Transform Cart Axis2/LConn1 -- Gyroscope/ Accelerometer/LConn1
  Transform Cart Axis4/RConn1 -- World Plane/RConn1
  Left Wheel/RConn1 -- Revolute Pendulum/RConn1
  Right Wheel/RConn1 -- Revolute Pendulum1/RConn1
  Spatial Contact Force1/LConn1 -- Spatial Contact Force/LConn1 -- World Plane/LConn1
  Mechanism Configuration/RConn1 -- Solver Configuration/RConn1 -- World Frame/RConn1 -- 6-DOF Joint/LConn1 -- Transform Cart Axis4/LConn1
  PS-Simulink Converter3/LConn1 -- Revolute Pendulum1/RConn2
  Revolute Pendulum1/RConn3 -- PS-Simulink Converter2/LConn1
  Simulink-PS Converter/RConn1 -- Revolute Pendulum/LConn2
  Revolute Pendulum/RConn3 -- PS-Simulink Converter/LConn1

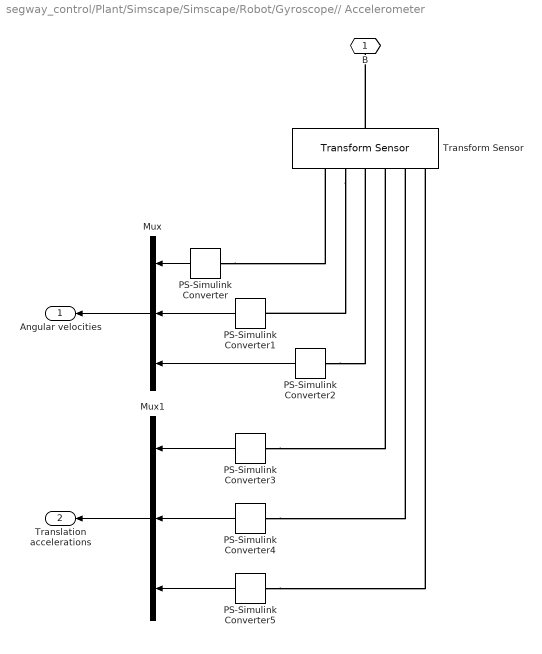
== system segway_control/Plant/Simscape/Simscape/Robot/Gyroscope// Accelerometer ==
  Mux : Mux  Inputs=3
  Mux1 : Mux  Inputs=3
  PS-Simulink Converter{,1..5} (6 alike) : nesl_utility/PS-Simulink Converter  PhysicalDomain=network_engine_domain  SubClassName=ps_output  LeftPortType=input  RightPortType=output  PseudoPeriodic=off  Frequencies=[]  VectorFormat=1-D array  Unit=1  AffineConversion=off
      settings: SourceProductBaseCode=PW,SS
  Transform Sensor : sm_lib/Frames and Transforms/Transform Sensor  MeasurementFrame=Base  SenseAngle=off  SenseAxis=off  SenseAngle1=off  SenseAngle2=off  SenseAngle3=off  SenseQ=off  SenseR=off  SenseOmegaX=on  SenseOmegaY=on  SenseOmegaZ=on  SenseOmega1=off  SenseOmega2=off  SenseOmega3=off  SenseQDot=off  SenseRDot=off  SenseAlphaX=off  SenseAlphaY=off  SenseAlphaZ=off  SenseAlpha1=off  SenseAlpha2=off  SenseAlpha3=off  SenseQDDot=off  SenseRDDot=off  SenseX=off  SenseY=off  SenseZ=off  SenseRad=off  SenseAzim=off  SenseDist=off  SenseInc=off  SenseXDot=off  SenseYDot=off  SenseZDot=off  SenseRadDot=off  SenseAzimDot=off  SenseDistDot=off  SenseIncDot=off  SenseXDDot=on  SenseYDDot=on  SenseZDDot=on  SenseRadDDot=off  SenseAzimDDot=off  SenseDistDDot=off  SenseIncDDot=off
  B : PMIOPort  Side=Left
  Angular velocities : Outport
  Translation accelerations : Outport  Port=2
  wires:
  PS-Simulink Converter4/1 -> Mux1/2
  PS-Simulink Converter5/1 -> Mux1/3
  Mux/1 -> Angular velocities/1
  PS-Simulink Converter1/1 -> Mux/2
  PS-Simulink Converter2/1 -> Mux/3
  PS-Simulink Converter3/1 -> Mux1/1
  Mux1/1 -> Translation accelerations/1
  PS-Simulink Converter/1 -> Mux/1
  connections:
  PS-Simulink Converter4/LConn1 -- Transform Sensor/RConn6
  Transform Sensor/RConn3 -- PS-Simulink Converter1/LConn1
  PS-Simulink Converter5/LConn1 -- Transform Sensor/RConn7
  PS-Simulink Converter2/LConn1 -- Transform Sensor/RConn4
  PS-Simulink Converter3/LConn1 -- Transform Sensor/RConn5
  Transform Sensor/LConn1 -- B/RConn1
  PS-Simulink Converter/LConn1 -- Transform Sensor/RConn2

== matlab function segway_control/Plant/Simscape/Simscape/MATLAB Function ==
  data: theta_l input; theta output; theta_r input
function theta = fcn(theta_l, theta_r)

theta = (theta_l + theta_r)/2;

== matlab function segway_control/Plant/Simscape/Simscape/MATLAB Function1 ==
  data: theta_l input; theta output; theta_r input
function theta = fcn(theta_l, theta_r)

theta = (theta_l + theta_r)/2;

== matlab function segway_control/Plant/Simscape/State Space1/get sensors ==
  data: enc_l output; enc_r output; y input; gyro output; R parameter; W parameter
function [enc_l, enc_r, gyro] = sensors(y, R, W)
enc_l = rad2deg(y(1) - W/R/2 * y(5) - y(2));
enc_r = rad2deg(y(1) + W/R/2 * y(5) - y(2));
gyro  = rad2deg(y(4));
